simulink model "RS232ex3"  (Simulink 8.7)
settings: Solver=ode3  StartTime=0.0  StopTime=10.0  FixedStep=0.01  RelTol=1e-3
libraries: RS232 x8
settings Model: Creator=Leonardo  LastModifiedBy=Leonardo
settings DataIOCC: SignalLoggingSaveFormat=ModelDataLogs  SignalLoggingName=sigsOut
settings OptimizationCC: BlockReduction=off  BooleanDataType=off
settings DebuggingCC: SaveWithParameterizedLinksMsg=none  SignalResolutionControl=TryResolveAllWithWarning  MultiTaskDSMMsg=warning  MultiTaskCondExecSysMsg=none
settings HardwareCC: TargetUnknown=on
settings GRTTargetCC: GeneratePreprocessorConditionals=Use local settings  CombineOutputUpdateFcns=off  GRTInterface=on

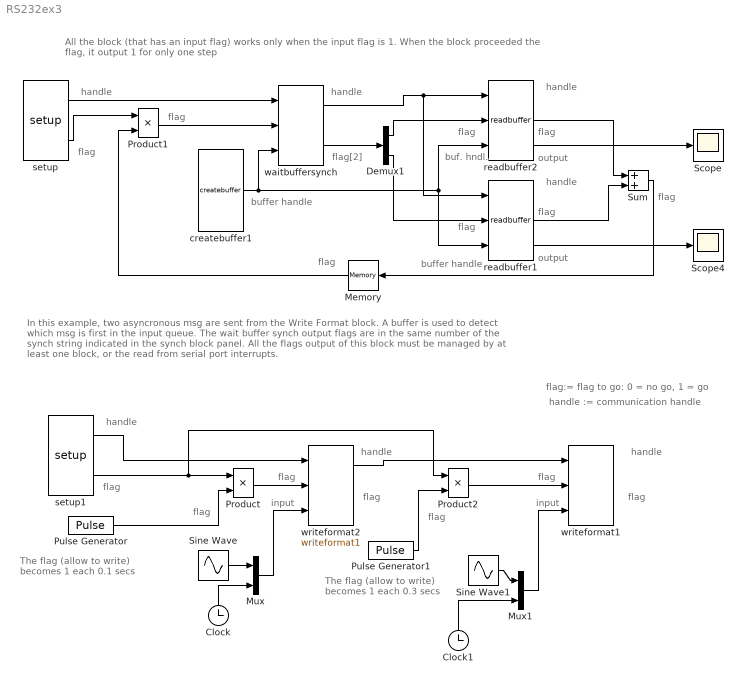
== system RS232ex3 ==
  note: handle
  note: handle
  note: handle
  note: handle
  note: handle
  note: handle
  note: handle
  note: buffer handle
  note: buffer handle
  note: buf. hndl.
  note: flag
  note: flag
  note: flag
  note: flag[2]
  note: flag
  note: flag
  note: flag
  note: flag
  note: flag
  note: flag
  note: flag
  note: flag
  note: flag
  note: flag
  note: flag
  note: flag
  note: output
  note: output
  note: input
  note: input
  note: In this example, two asyncronous msg are sent from the Write Format block. A buffer is used to detect which msg is first in the input queue.
      | The wait buffer synch output flags are in the same number of the synch string indicated in the synch block panel. All the flags output of this block
      | must be managed by at least one block, or the read from serial port interrupts.
  note: The flag (allow to write)
      | becomes 1 each 0.1 secs
  note: The flag (allow to write)
      | becomes 1 each 0.3 secs
  note: All the block (that has an input flag) works only when the input flag is 1. When the block proceeded the flag, it output 1 for only one step
  note: flag:= flag to go: 0 = no go, 1 = go
  note: handle := communication handle
  Clock : Clock
  Clock1 : Clock
  Demux1 : Demux  Outputs=2
  Memory : Memory  X0=1
  Mux : Mux  Inputs=2
  Mux1 : Mux  Inputs=2
  Product : Product  SaturateOnIntegerOverflow=on  OutDataTypeStr=Inherit: Same as first input
  Product1 : Product  SaturateOnIntegerOverflow=on  OutDataTypeStr=Inherit: Same as first input
  Product2 : Product  SaturateOnIntegerOverflow=on  OutDataTypeStr=Inherit: Same as first input
  Pulse Generator : DiscretePulseGenerator  PulseType=Time based  Period=0.1  PulseWidth=10
  Pulse Generator1 : DiscretePulseGenerator  PulseType=Time based  Period=0.3  PulseWidth=10
  Scope : Scope
  Scope4 : Scope
  Sine Wave : Sin  SampleTime=0.01
  Sine Wave1 : Sin  Frequency=2  Phase=90  SampleTime=0.01
  Sum : Sum  SaturateOnIntegerOverflow=on
  createbuffer1 : RS232/createbuffer  minbuffsize=128  sampletime=-1
  readbuffer1 : RS232/readbuffer  fmtString=msg2;%f,%f;end  nCharTerm=4  sampTime=-1  allocstep=128
  readbuffer2 : RS232/readbuffer  fmtString=msg1;%f,%f\r\n  nCharTerm=2  sampTime=-1  allocstep=128
  setup : RS232/setup  port=COM2  baudrate=460800  databit=8  stopbit=1  parity=None
  setup1 : RS232/setup  port=COM3  baudrate=460800  databit=8  stopbit=1  parity=None
  waitbuffersynch : RS232/waitbuffersynch  synchString=msg1;, msg2;  sampTime=-1  allocstep=128
  writeformat1 : RS232/writeformat1  fmtString=msg2;%f,%f;end  sampTime=-1
  writeformat2 : RS232/writeformat1  fmtString=msg1;%f,%f\r\n  sampTime=-1
  wires:
  setup/1 -> waitbuffersynch/1
  setup/2 -> Product1/1
  createbuffer1/1 -> readbuffer2/3, readbuffer1/3, waitbuffersynch/3
  waitbuffersynch/1 -> readbuffer2/1, readbuffer1/1
  readbuffer2/2 -> Sum/1
  Memory/1 -> Product1/2
  Product1/1 -> waitbuffersynch/2
  waitbuffersynch/2 -> Demux1/1
  Demux1/1 -> readbuffer2/2
  setup1/1 -> writeformat2/1
  setup1/2 -> Product/1, Product2/1
  Clock/1 -> Mux/2
  Sine Wave/1 -> Mux/1
  Mux/1 -> writeformat2/3
  Pulse Generator/1 -> Product/2
  Product/1 -> writeformat2/2
  writeformat2/1 -> writeformat1/1
  Sine Wave1/1 -> Mux1/1
  Clock1/1 -> Mux1/2
  Mux1/1 -> writeformat1/3
  Pulse Generator1/1 -> Product2/2
  Product2/1 -> writeformat1/2
  Demux1/2 -> readbuffer1/2
  readbuffer1/3 -> Scope4/1
  readbuffer1/2 -> Sum/2
  Sum/1 -> Memory/1
  readbuffer2/3 -> Scope/1
